simulink model "shem4"  (R2023a)
settings: Solver=VariableStepAuto  StartTime=0.0  StopTime=10.0  RelTol=1e-3
libraries: simulink x4
settings Model: Creator=fynjy  LastModifiedBy=fynjy

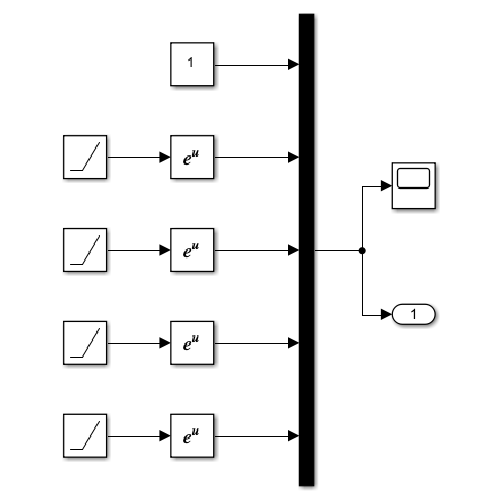
[thumbnail: Simulink's stored preview of the top-level diagram]
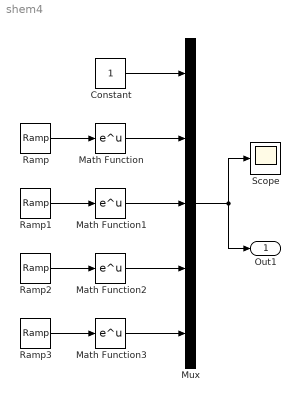
== system shem4 ==
  Constant : Constant
  Math Function{,1..3} (4 alike) : Math
  Mux : Mux  Inputs=5
  Ramp{,1..3} (4 alike) : simulink/Sources/Ramp  slope=1  start=0  InitialOutput=0
  Scope : Scope
  Out1 : Outport
  wires:
  Mux/1 -> Out1/1, Scope/1
  Ramp2/1 -> Math Function2/1
  Ramp3/1 -> Math Function3/1
  Ramp1/1 -> Math Function1/1
  Ramp/1 -> Math Function/1
  Constant/1 -> Mux/1
  Math Function/1 -> Mux/2
  Math Function1/1 -> Mux/3
  Math Function2/1 -> Mux/4
  Math Function3/1 -> Mux/5
